simulink model "TestPathFollowing1"  (R2022a)
settings: Solver=VariableStepAuto  StartTime=0.0  StopTime=2000  RelTol=1e-3
libraries: mssSimulink x3
settings Model: Creator=Lenovo  LastModifiedBy=Lenovo

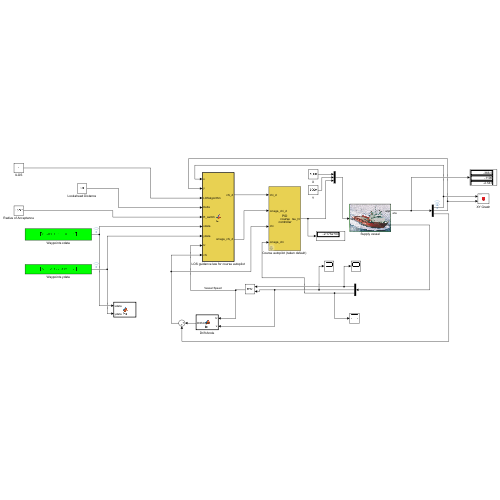
[thumbnail: Simulink's stored preview of the top-level diagram]
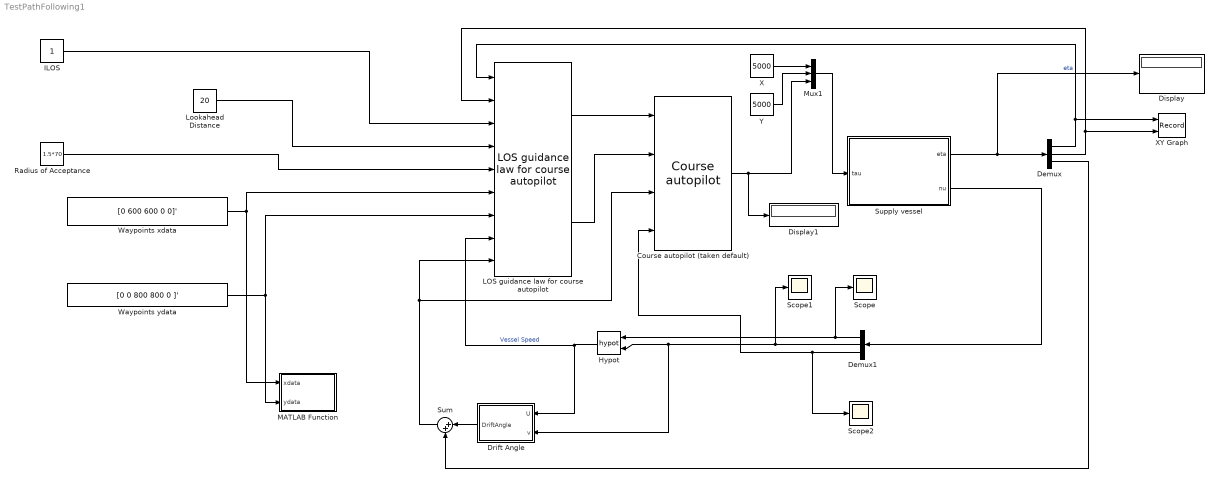
== system TestPathFollowing1 ==
  "Course autopilot (taken default) " : mssSimulink/Control/Autopilots/Course autopilot  wn=1.2  zeta=1  T_nomoto=0.5  m=37.5
  Demux : Demux  Outputs=3
  Demux1 : Demux  Outputs=3
  Display : Display
  Display1 : Display
  Drift Angle : MATLAB Function  TreatAsAtomicUnit=on
  Hypot : Math  Operator=hypot
  ILOS : Constant
  LOS guidance law for course autopilot : mssSimulink/Guidance/LOS guidance law for course autopilot  SystemSampleTime=-1  VariantActivationTime=update diagram  Latency=0  AutoFrameSizeCalculation=off
  Lookahead Distance : Constant  Value=20
  MATLAB Function : MATLAB Function  TreatAsAtomicUnit=on
  Mux1 : Mux  Inputs=3
  Radius of Acceptance : Constant  Value=1.5*70
  Scope : Scope
  Scope1 : Scope
  Scope2 : Scope
  Sum : Sum  Inputs=|++
  Supply vessel : Subsystem  AncestorBlock=mssSimulink/Marine craft models/Supply vessel  mask(Supply Vessel (surge, sway and yaw)){D=[5.0242e4 0 0; 0 2.7229e5 -4.3933e6; 0 -4.3933e6 4.1894e8], Minv=inv( [5.3122e6 0 0; 0 8.2831e6 0; 0 0 3.7454e9] )}
      mask prompts: D "Linear damping matrix: D"; Minv "Inverse inertia matrix: Minv"
      mask help:
      | DP model
      |
      | Inputs:
      |
      |    tau = 3 DOF control input vector (generalized force)
      |
      | Outputs:
      |
      |    eta = [x, y, psi]'
      |    nu  = [u, v, r]'
      mask Display:
      | image(imread('simulink/figs/supply.jpg'))
      | color('black'); port_label('output', 1, 'eta')
      | color('black'); port_label('output', 2, 'nu')
      | color('black'); port_label('input', 1, 'tau')
  Waypoints xdata : Constant  Value=[0 600 600 0 0]'
  Waypoints ydata : Constant  Value=[0 0 800 800 0 ]'
  X : Constant  Value=5000
  XY Graph : Record  FileSettingsInternal="{\"entries\":[{\"content\":{\"excelSettings\":{\"content\":{},\"type\":\"Streamout.ExcelSettings\"}},\"type\":\"Streamout.FileSettingStorage\",\"uuid\":\"e9fc0062-165c-4f03-98dc-a1043815026f\"}],\"packageUris\":[\"http://schema.mathworks.com/mf0/streamout_blocks/R2020a\"],\"version\":\"1.0\"}"  Layout=[1 1]  SignalsInternal="{\"entries\":[{\"content\":{\"signals\":[{\"content\":{\"blockPath\":[\"untitled/XY Graph\"],\"channel\":[],\"dimensions\":[1],\"domain\":\"untitled/XY Graph\",\"lineColor\":\"#a2142f\",\"plots\":[1],\"port\":1,\"sid\":[\"\"],\"signalID\":4678,\"signalName\":\"Demux:1\"},\"type\":\"RecordBlkView.Signal\",\"uuid\":\"7d965e95-9cd0-4d65-a421-d29a657c3667\"},{\"content\":{\"blockPath\":[\"untitled/XY Graph\"],\"channel\":[],\"dimensions\":[1],\"domain\":\"untitled/XY Graph\",\"lineColor\":\"#139fff\",\"plots\":[1],\"port\":2,\"sid\":[\"\"],\"signalID\":4682,\"signalName\":\"Demux:2\"},\"type\":\"RecordBlkView.Signal\",\"uuid\":\"efd6257d-5c6c-4a8f-ab0c-ff8ee1b65cc7\"}]},\"type\":\"RecordBlkView.InputSignals\",\"uuid\":\"98f75197-0b0f-4e46-9333-0df6d149553c\"}],\"packageUris\":[\"http://schema.mathworks.com/mf0/streamout_blocks/R2020a\"],\"version\":\"1.0\"}"  VisualizationBindings="{\"xyplotplugin\":{\"info\":[{\"series\":[{\"bindingParametersList\":[{\"parameter\":\"X-Axis\",\"signalID\":4678,\"signalName\":\"Demux:1\"},{\"parameter\":\"Y-Axis\",\"signalID\":4682,\"signalName\":\"Demux:2\"}],\"seriesID\":35066}],\"subplotID\":1}]}}"  CompatibilityTag=XY
  Y : Constant  Value=5000
  wires:
  LOS guidance law for course autopilot/1 -> "Course autopilot (taken default) "/1
  LOS guidance law for course autopilot/2 -> "Course autopilot (taken default) "/2
  Supply vessel/1(eta) -> Display/1, Demux/1  "eta"
  Demux/1 -> XY Graph/1, LOS guidance law for course autopilot/1
  Demux/2 -> XY Graph/2, LOS guidance law for course autopilot/2
  ILOS/1 -> LOS guidance law for course autopilot/3
  Waypoints xdata/1 -> MATLAB Function/1(xdata), LOS guidance law for course autopilot/6
  Waypoints ydata/1 -> MATLAB Function/2(ydata), LOS guidance law for course autopilot/7
  Radius of Acceptance/1 -> LOS guidance law for course autopilot/5
  Supply vessel/2(nu) -> Demux1/1
  Demux1/1 -> Scope/1, Hypot/1
  Demux1/2 -> Scope1/1, Drift Angle/2(v), Hypot/2
  Hypot/1 -> Drift Angle/1(U), LOS guidance law for course autopilot/8  "Vessel Speed"
  Demux/3 -> Sum/2
  Drift Angle/1(DriftAngle) -> Sum/1
  Sum/1 -> LOS guidance law for course autopilot/9, "Course autopilot (taken default) "/3
  Demux1/3 -> Scope2/1, "Course autopilot (taken default) "/4
  Lookahead Distance/1 -> LOS guidance law for course autopilot/4
  X/1 -> Mux1/1
  Y/1 -> Mux1/2
  "Course autopilot (taken default) "/1 -> Display1/1, Mux1/3
  Mux1/1 -> Supply vessel/1(tau)

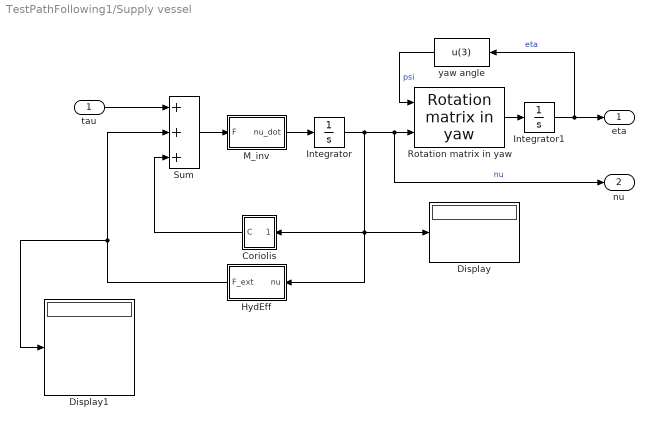
== system TestPathFollowing1/Supply vessel ==
  tau : Inport
  Coriolis : Subsystem
  Display : Display
  Display1 : Display
  HydEff : Subsystem
  Integrator : Integrator  InitialCondition=[0 1 0]
  Integrator1 : Integrator
  M_inv : Subsystem
  "Rotation matrix in yaw " : mssSimulink/Modelling/Kinematics/Rotation matrix in yaw 
  Sum : Sum  Inputs=+++  InputSameDT=on  SaturateOnIntegerOverflow=on  OutDataTypeStr=Inherit: Same as first input
  yaw angle : Fcn  Expr=u(3)
  eta : Outport  InitialOutput=0  VectorParamsAs1DForOutWhenUnconnected=off
  nu : Outport  Port=2  InitialOutput=0  VectorParamsAs1DForOutWhenUnconnected=off
  wires:
  Sum/1 -> M_inv/1(F)
  M_inv/1(nu_dot) -> Integrator/1
  tau/1 -> Sum/1
  "Rotation matrix in yaw "/1 -> Integrator1/1
  yaw angle/1 -> "Rotation matrix in yaw "/1  "psi"
  Integrator/1 -> Display/1, HydEff/1(nu), Coriolis/1(nu), "Rotation matrix in yaw "/2, nu/1  "nu"
  Integrator1/1 -> yaw angle/1, eta/1  "eta"
  HydEff/1(F_ext) -> Display1/1, Sum/2
  Coriolis/1(C) -> Sum/3

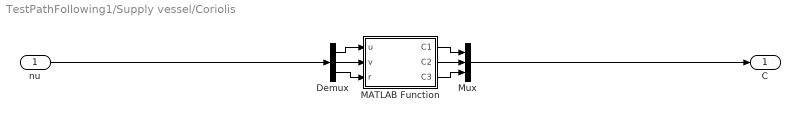
== system TestPathFollowing1/Supply vessel/Coriolis ==
  nu : Inport
  Demux : Demux  Outputs=3
  MATLAB Function : MATLAB Function  TreatAsAtomicUnit=on
  Mux : Mux  Inputs=3
  C : Outport
  wires:
  nu/1 -> Demux/1
  MATLAB Function/2(C2) -> Mux/2
  MATLAB Function/3(C3) -> Mux/3
  MATLAB Function/1(C1) -> Mux/1
  Mux/1 -> C/1
  Demux/1 -> MATLAB Function/1(u)
  Demux/2 -> MATLAB Function/2(v)
  Demux/3 -> MATLAB Function/3(r)

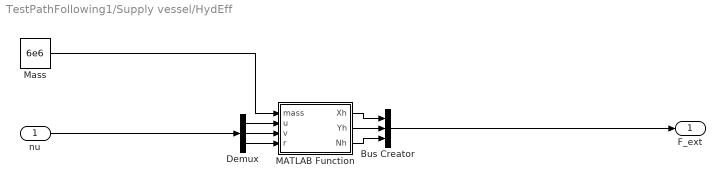
== system TestPathFollowing1/Supply vessel/HydEff ==
  nu : Inport
  Bus Creator : BusCreator  Inputs=3
  Demux : Demux  Outputs=3
  MATLAB Function : MATLAB Function  TreatAsAtomicUnit=on
  Mass : Constant  Value=6e6
  F_ext : Outport
  wires:
  Mass/1 -> MATLAB Function/1(mass)
  MATLAB Function/1(Xh) -> Bus Creator/1
  Bus Creator/1 -> F_ext/1
  MATLAB Function/2(Yh) -> Bus Creator/2
  MATLAB Function/3(Nh) -> Bus Creator/3
  nu/1 -> Demux/1
  Demux/1 -> MATLAB Function/2(u)
  Demux/2 -> MATLAB Function/3(v)
  Demux/3 -> MATLAB Function/4(r)

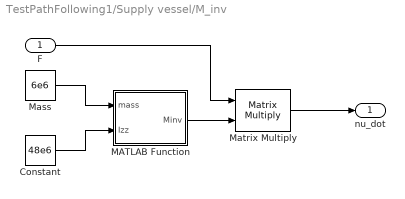
== system TestPathFollowing1/Supply vessel/M_inv ==
  F : Inport
  Constant : Constant  Value=48e6
  MATLAB Function : MATLAB Function  TreatAsAtomicUnit=on
  Mass : Constant  Value=6e6
  Matrix Multiply : Product  Multiplication=Matrix(*)
  nu_dot : Outport
  wires:
  MATLAB Function/1(Minv) -> Matrix Multiply/2
  Mass/1 -> MATLAB Function/1(mass)
  Constant/1 -> MATLAB Function/2(Izz)
  Matrix Multiply/1 -> nu_dot/1
  F/1 -> Matrix Multiply/1

== matlab function TestPathFollowing1/Supply vessel/Coriolis/MATLAB Function ==
  data: u input; C1 output; C2 output; C3 output; v input; r input
function [C1,    C2,    C3]    = fcn(u,v,r)

% u = nu(1);
% v = nu(2);
% r = nu(3);

x_g = 0;
m = 6e6;

C = [0                 0  -m*(x_g*r + v); ...
     0                 0             m*u; ...
     m*(x_g*r + v)  -m*u              0];

Co = C*[u;v;r];
C1 = Co(1);
C2 = Co(2);
C3 = Co(3);

end

== matlab function TestPathFollowing1/Drift Angle ==
  data: U input; DriftAngle output; v input
function DriftAngle = fcn(U,v)

    DriftAngle = asin(v/U);
end

== matlab function TestPathFollowing1/Supply vessel/M_inv/MATLAB Function ==
  data: Minv output; mass input; Izz input
function Minv = fcn(mass, Izz)

h.m   = mass;    % Mass [Kg]
h.Izz = Izz;     % Yaw Inertia
h.xG  = 0;

%%%%%%%%%%%%%%%%%%%%%%%%%%%%%%%%%%%%%%%%%%%%%%%%%%%%%%%%%%%%%%%%%%%%%%%
% The hydrodynamic derivatives are given in dimensional form, and follow
% from the original publication of Blanke and Christensen 1993.
%%%%%%%%%%%%%%%%%%%%%%%%%%%%%%%%%%%%%%%%%%%%%%%%%%%%%%%%%%%%%%%%%%%%%%%
% Data for surge equation 
h.Xudot  	= -17400.0;
h.Xuau     	= -1.96e+003;
h.Xvr    	=  0.33 * mass;
   
% Hydrodynamic coefficients in sway equation
h.Yvdot = -393000; 
h.Ypdot = -296000; 
h.Yrdot = -1400000; 
h.Yauv  = -11800; 
h.Yur   =  131000; 
h.Yvav  = -3700; 
h.Yrar  =  0;
h.Yvar  = -794000; 
h.Yrav  = -182000; 
h.Ybauv =  10800; % Y_{\phi |v u|}
h.Ybaur =  251000; 
h.Ybuu  = -74;


% Hydrodynamic coefficients in yaw equation
h.Nvdot =  538000;
h.Npdot =  0;
h.Nrdot = -38.7e6;
h.Nauv  = -92000;
h.Naur  = -4710000;
h.Nvav  =  0;
h.Nrar  = -202000000;
h.Nvar  =  0;
h.Nrav  = -15600000;
h.Nbauv = -214000;
h.Nbuar = -4980000;
h.Nbuau = -8000;
%%%%%%%%%%%%%%%%%%%%%%%%%%%%%%%%%%%%%%%%%%%%%%%%%%%%%%%%%%%%%%%%%%%%%%%%%%%


M = [(h.m-h.Xudot)                  0                  0; ...
                 0      (h.m-h.Yvdot) (h.m*h.xG-h.Yrdot); ...
                 0 (h.m*h.xG-h.Nvdot)    (h.Izz-h.Nrdot)];

Minv = inv(M);
end

== matlab function TestPathFollowing1/Supply vessel/HydEff/MATLAB Function ==
  data: mass input; Xh output; Yh output; Nh output; u input; v input; r input
function [Xh, Yh, Nh] = fcn(mass, u, v, r)

%%%%%%%%%%%%%%%%%%%%%%%%%%%%%%%%%%%%%%%%%%%%%%%%%%%%%%%%%%%%%%%%%%%%%%%
% The hydrodynamic derivatives are given in dimensional form, and follow
% from the original publication of Blanke and Christensen 1993.
%%%%%%%%%%%%%%%%%%%%%%%%%%%%%%%%%%%%%%%%%%%%%%%%%%%%%%%%%%%%%%%%%%%%%%%
% Data for surge equation 
h.Xudot  	= -17400.0 ;
h.Xuau     	= -1.96e+003 ;
h.Xvr    	=  0.33 * mass ;
   
% Hydrodynamic coefficients in sway equation
h.Yvdot = -393000 ; 
h.Ypdot = -296000 ; 
h.Yrdot = -1400000 ; 
h.Yauv  = -11800 ; 
h.Yur   =  131000 ; 
h.Yvav  = -3700 ; 
h.Yrar   =  0 ;
h.Yvar  = -794000 ; 
h.Yrav  = -182000 ; 
h.Ybauv =  10800 ; % Y_{\phi |v u|}
h.Ybaur =  251000 ; 
h.Ybuu  = -74 ; 


% Hydrodynamic coefficients in yaw equation
h.Nvdot =  538000 ;
h.Npdot =  0 ;
h.Nrdot = -38.7e6;
h.Nauv  = -92000 ;
h.Naur  = -4710000 ;
h.Nvav  =  0 ;
h.Nrar  = -202000000 ;
h.Nvar  =  0 ;
h.Nrav  = -15600000 ;
h.Nbauv = -214000 ;
h.Nbuar = -4980000 ;
h.Nbuau = -8000 ;
%%%%%%%%%%%%%%%%%%%%%%%%%%%%%%%%%%%%%%%%%%%%%%%%%%%%%%%%%%%%%%%%%%%%%%%%%%%

au = abs(u);
av = abs(v); 
ar = abs(r);
b = 0;

% Hydrodynamic forces without added mass terms (considered in the M matrix)
Xh  = h.Xuau*u*au+h.Xvr*v*r;

Yh = h.Yauv*au*v + h.Yur*u*r + h.Yvav*v*av + h.Yvar*v*ar + h.Yrav*r*av ...
   + h.Ybauv*b*abs(u*v) + h.Ybaur*b*abs(u*r) + h.Ybuu*b*u^2;

Nh = h.Nauv*au*v + h.Naur*au*r + h.Nrar*r*ar + h.Nrav*r*av...
   +h.Nbauv*b*abs(u*b) + h.Nbuar*b*u*ar + h.Nbuau*b*u*au;

end

== matlab function TestPathFollowing1/MATLAB Function ==
  data: xdata input; ydata input
function  fcn(xdata, ydata)

 plot(xdata,ydata);
 axis([-200 800 -300 1000])
 
end
